simulink model "week1prob1"  (R2020b)
settings: Solver=VariableStepAuto  StartTime=0.0  StopTime=10.0  RelTol=1e-3
model workspace (MAT data in the model file):
  K1 = Simulink.Parameter
  K1.Value = 50
  K1.DataType = 'auto'
  K1.Dimensions = [1 1]
  M1 = Simulink.Parameter
  M1.Value = 100
  M1.DataType = 'auto'
  M1.Dimensions = [1 1]
  M2 = Simulink.Parameter
  M2.Value = 20
  M2.DataType = 'auto'
  M2.Dimensions = [1 1]
  b = Simulink.Parameter
  b.Value = 50
  b.DataType = 'auto'
  b.Dimensions = [1 1]
  omega = Simulink.Parameter
  omega.Value = 10
  omega.DataType = 'auto'
  omega.Dimensions = [1 1]
settings Model: Creator=lalit  LastModifiedBy=lalit

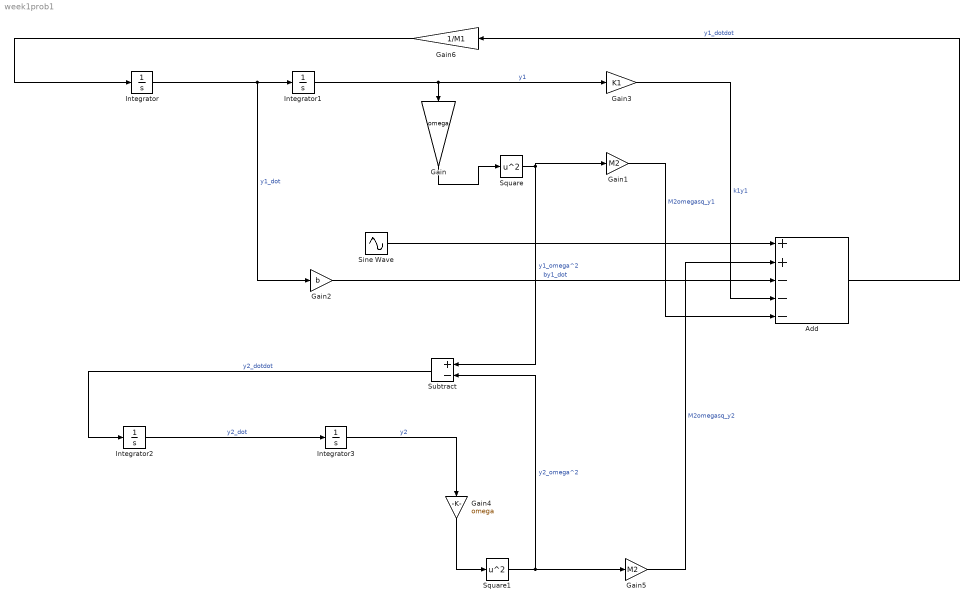
== system week1prob1 ==
  Add : Sum  Inputs=++---
  Gain : Gain  Gain=omega
  Gain1 : Gain  Gain=M2
  Gain2 : Gain  Gain=b
  Gain3 : Gain  Gain=K1
  Gain4 : Gain  Gain=omega
  Gain5 : Gain  Gain=M2
  Gain6 : Gain  Gain=1/M1
  Integrator{,1..3} (4 alike) : Integrator
  Sine Wave : Sin  Amplitude=2  Frequency=10  SampleTime=0
  Square : Math  Operator=square  SaturateOnIntegerOverflow=on
  Square1 : Math  Operator=square  SaturateOnIntegerOverflow=on
  Subtract : Sum  Inputs=+-
  wires:
  Integrator/1 -> Gain2/1, Integrator1/1  "y1_dot"
  Integrator2/1 -> Integrator3/1  "y2_dot"
  Integrator1/1 -> Gain3/1, Gain/1  "y1"
  Subtract/1 -> Integrator2/1  "y2_dotdot"
  Integrator3/1 -> Gain4/1  "y2"
  Gain/1 -> Square/1
  Square/1 -> Gain1/1, Subtract/1  "y1_omega^2"
  Gain1/1 -> Add/5  "M2omegasq_y1"
  Gain3/1 -> Add/4  "k1y1"
  Sine Wave/1 -> Add/1
  Gain2/1 -> Add/3  "by1_dot"
  Add/1 -> Gain6/1  "y1_dotdot"
  Gain4/1 -> Square1/1
  Gain5/1 -> Add/2  "M2omegasq_y2"
  Square1/1 -> Subtract/2, Gain5/1  "y2_omega^2"
  Gain6/1 -> Integrator/1
